simulink model "neuronchainv6"  (Simulink 7.6)
settings: Solver=ode45  StartTime=0.0  StopTime=300  RelTol=1e-3
values from neighbouring files (symbols this model uses):
  alpha = 0.8    [excneuroninit.m]
  beta = 0.05    [excneuroninit.m]
  inittime = 0.1    [excneuroninit.m]
  sensoryamp = 0.5    [excneuroninit.m]
  sigslopef = 1    [excneuroninit.m]
  sigslopei = 3    [excneuroninit.m]
  tau_s = 5    [excneuroninit.m]
libraries: simulink x500, neuronpoolibv3 x3
(part 1 of 18)
settings Model: Creator=root  LastModifiedBy=root
settings SolverCC: ZeroCrossAlgorithm=Adaptive

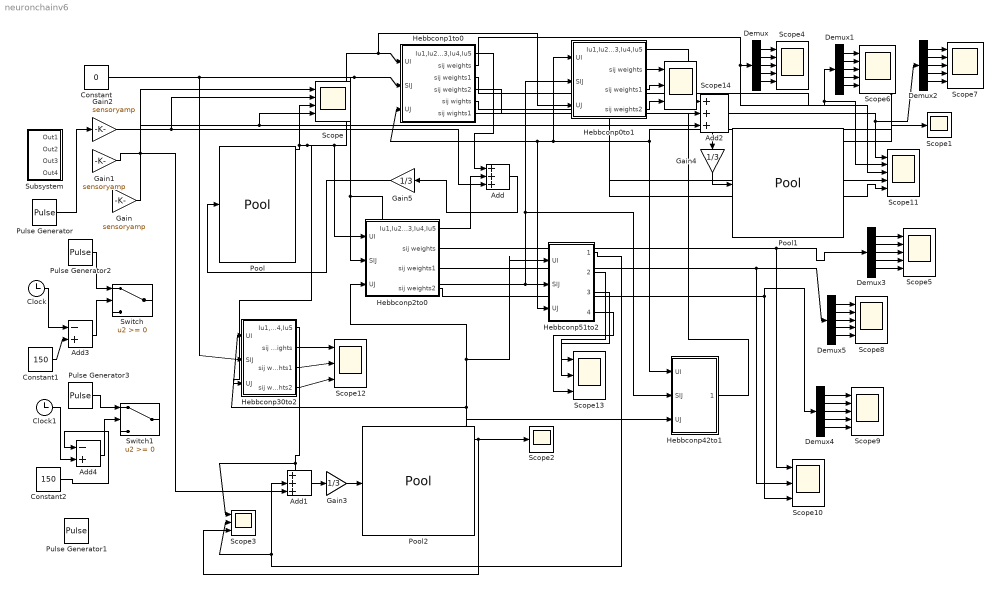
== system neuronchainv6 ==
  Add : Sum  Inputs=+++
  Add1 : Sum  Inputs=+++
  Add2 : Sum  Inputs=+++
  Add3 : Sum  Inputs=-+
  Add4 : Sum  Inputs=-+
  Clock : Clock
      settings: Decimation=10
  Clock1 : Clock
      settings: Decimation=10
  Constant : Constant  Value=0
  Constant1 : Constant  Value=150
  Constant2 : Constant  Value=150
  Demux{,1..5} (6 alike) : Demux  Outputs=5
  Gain : Gain  Gain=sensoryamp
  Gain1 : Gain  Gain=sensoryamp
  Gain2 : Gain  Gain=sensoryamp
  Gain3 : Gain  Gain=1/3
  Gain4 : Gain  Gain=1/3
  Gain5 : Gain  Gain=1/3
  Hebbconp0to1 : Subsystem
  Hebbconp1to0 : Subsystem
  Hebbconp2to0 : Subsystem
  Hebbconp30to2 : Subsystem
  Hebbconp42to1 : Subsystem
  Hebbconp51to2 : Subsystem
  Pool : neuronpoolibv3/Pool  SystemSampleTime=-1
  Pool1 : neuronpoolibv3/Pool  SystemSampleTime=-1
  Pool2 : neuronpoolibv3/Pool  SystemSampleTime=-1
  Pulse Generator : DiscretePulseGenerator  PulseType=Time based  Period=1  PulseWidth=50
  Pulse Generator1 : DiscretePulseGenerator  PulseType=Time based  Period=1  PulseWidth=50  PhaseDelay=0.5
  Pulse Generator2 : DiscretePulseGenerator  PulseType=Time based  PulseWidth=25  PhaseDelay=1.35
  Pulse Generator3 : DiscretePulseGenerator  PulseType=Time based  PulseWidth=25  PhaseDelay=1.35
  Scope : Scope  NumInputPorts=4
      settings: TimeRange=100  YMin=-1~0~3.9~-1  YMax=1~0.5~4.3~1
  Scope1 : Scope
      settings: YMin=6.5  YMax=12.25
  Scope{3,10,12..14} (5 alike) : Scope  NumInputPorts=3
      Scope10 settings: YMin=0.0405~0.04075~0.04075  YMax=0.0435~0.04375~0.044  SaveName=ScopeData10
      Scope12 settings: YMin=0.3~0.3~0.3  YMax=0.75~0.7~0.7  SaveName=ScopeData12
      Scope13 settings: YMin=0.06~0.06~0.06  YMax=0.15~0.14~0.14  SaveName=ScopeData13
      Scope14 settings: TimeRange=300  YMin=0.166~0.1635~0.1625  YMax=0.1715~0.169~0.1675  SaveName=ScopeData14
      Scope3 settings: YMin=3.46~3.4525~3.9  YMax=3.51~3.4825~4.1  SaveName=ScopeData3
  Scope{4..9,11} (7 alike) : Scope  NumInputPorts=5
      Scope11 settings: YMin=0.0053~0.0054~0.0054~-5~-5  YMax=0.0064~0.0065~0.0065~5~5  SaveName=ScopeData11
      Scope4 settings: YMin=0.177~0.162~0.1565~0.162~0.177  YMax=0.183~0.166~0.1605~0.166~0.183  SaveName=ScopeData4
      Scope5 settings: YMin=0.177~0.162~0.1565~0.162~0.177  YMax=0.183~0.166~0.1605~0.166~0.183  SaveName=ScopeData5
      Scope6 settings: YMin=0.567164~0.567164~0.567164~-5~-5  YMax=0.626866~0.626866~0.626866~5~5  SaveName=ScopeData6
      Scope7 settings: YMin=0.567164~0.567164~0.567164~-5~-5  YMax=0.626866~0.626866~0.626866~5~5  SaveName=ScopeData7
      Scope8 settings: YMin=0.171~0.14425~0.13725~0.14425~0.171  YMax=0.175~0.14625~0.13925~0.14625~0.175  SaveName=ScopeData8
      Scope9 settings: YMin=0.06~0.06~0.06~0.06~0.06  YMax=0.15~0.14~0.14~0.14~0.15  SaveName=ScopeData9
  Scope2 : Scope
      settings: SaveName=ScopeData2
  Subsystem : Subsystem
  Switch : Switch
  Switch1 : Switch
  wires:
  Pool/1 -> Hebbconp1to0/1(UI), Hebbconp0to1/3(UJ), Hebbconp2to0/1(UI), Hebbconp30to2/3(UJ), Scope/3
  Pool1/1 -> Hebbconp1to0/3(UJ), Hebbconp51to2/3(UJ), Hebbconp0to1/1(UI), Hebbconp42to1/1(UI), Scope1/1
  Pool2/1 -> Hebbconp2to0/3(UJ), Hebbconp51to2/1(UI), Hebbconp30to2/1(UI), Hebbconp42to1/3(UJ), Scope2/1, Scope3/3
  Hebbconp1to0/1(Iu1,Iu2,Iu3,Iu4,Iu5) -> Add/1
  Add/1 -> Gain5/1
  Hebbconp51to2/1(Iu1,Iu2,Iu3,Iu4,Iu5) -> Add1/2, Scope3/2
  Hebbconp30to2/1(Iu1,Iu2,Iu3,Iu4,Iu5) -> Add1/1, Scope3/1
  Add1/1 -> Gain3/1
  Hebbconp42to1/1(Iu1,Iu2,Iu3,Iu4,Iu5) -> Add2/2
  Add2/1 -> Gain4/1
  Constant/1 -> Hebbconp1to0/2(SIJ), Hebbconp42to1/2(SIJ), Hebbconp0to1/2(SIJ), Hebbconp51to2/2(SIJ), Hebbconp2to0/2(SIJ), Hebbconp30to2/2(SIJ)
  Hebbconp2to0/1(Iu1,Iu2,Iu3,Iu4,Iu5) -> Add/2
  Hebbconp2to0/2(sij weights) -> Demux3/1, Scope10/1
  Hebbconp2to0/3(sij weights1) -> Demux5/1, Scope10/2
  Hebbconp2to0/4(sij weights2) -> Demux4/1, Scope10/3
  Gain/1 -> Add2/3, Scope/4
  Gain1/1 -> Add1/3, Scope/1
  Gain2/1 -> Add/3, Scope/2
  Demux/1 -> Scope4/1
  Demux/2 -> Scope4/2
  Demux/3 -> Scope4/3
  Demux/4 -> Scope4/4
  Demux/5 -> Scope4/5
  Hebbconp1to0/2(sij weights) -> Demux/1, Scope11/3
  Demux1/1 -> Scope6/1
  Demux1/2 -> Scope6/2
  Demux1/3 -> Scope6/3
  Demux1/4 -> Scope6/4
  Demux1/5 -> Scope6/5
  Hebbconp1to0/3(sij weights1) -> Demux1/1, Scope11/2
  Demux2/1 -> Scope7/1
  Demux2/2 -> Scope7/2
  Demux2/3 -> Scope7/3
  Demux2/4 -> Scope7/4
  Demux2/5 -> Scope7/5
  Hebbconp1to0/4(sij weights2) -> Demux2/1, Scope11/1
  Demux5/1 -> Scope8/1
  Demux5/2 -> Scope8/2
  Demux5/3 -> Scope8/3
  Demux5/4 -> Scope8/4
  Demux5/5 -> Scope8/5
  Demux3/1 -> Scope5/1
  Demux3/2 -> Scope5/2
  Demux3/3 -> Scope5/3
  Demux3/4 -> Scope5/4
  Demux3/5 -> Scope5/5
  Demux4/1 -> Scope9/1
  Demux4/2 -> Scope9/2
  Demux4/3 -> Scope9/3
  Demux4/4 -> Scope9/4
  Demux4/5 -> Scope9/5
  Hebbconp1to0/5(sij wights) -> Scope11/4
  Hebbconp1to0/6(sij wights1) -> Scope11/5
  Hebbconp30to2/2(sij weights) -> Scope12/1
  Hebbconp30to2/3(sij weights1) -> Scope12/2
  Hebbconp30to2/4(sij weights2) -> Scope12/3
  Hebbconp51to2/2(sij weights) -> Scope13/1
  Hebbconp51to2/3(sij weights1) -> Scope13/2
  Hebbconp51to2/4(sij weights2) -> Scope13/3
  Hebbconp0to1/1(Iu1,Iu2,Iu3,Iu4,Iu5) -> Add2/1
  Hebbconp0to1/2(sij weights) -> Scope14/1
  Hebbconp0to1/3(sij weights1) -> Scope14/2
  Hebbconp0to1/4(sij weights2) -> Scope14/3
  Gain5/1 -> Pool/1
  Gain3/1 -> Pool2/1
  Gain4/1 -> Pool1/1
  Clock/1 -> Add3/1
  Constant1/1 -> Add3/2
  Add3/1 -> Switch/2
  Pulse Generator/1 -> Gain2/1
  Add4/1 -> Switch1/2
  Clock1/1 -> Add4/2
  Constant2/1 -> Add4/1
  Pulse Generator2/1 -> Switch/1
  Pulse Generator3/1 -> Switch1/1

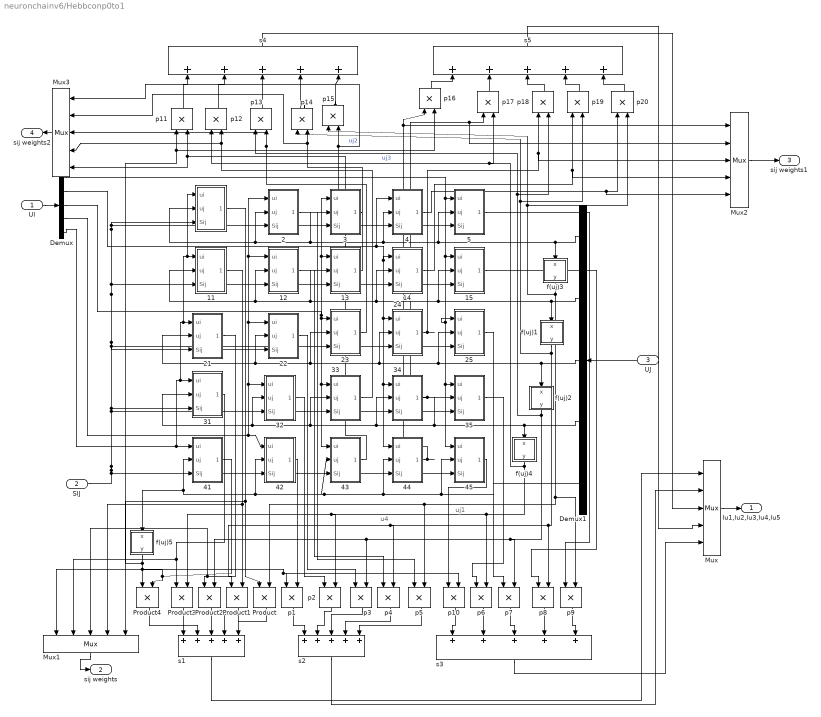
== system neuronchainv6/Hebbconp0to1 ==
  note: uj1
  note: u4
  UI : Inport
  SIJ : Inport  Port=2
  UJ : Inport  Port=3
  " " : Subsystem
  " 2" : Subsystem
  11 : Subsystem
  12 : Subsystem
  13 : Subsystem
  14 : Subsystem
  15 : Subsystem
  21 : Subsystem
  22 : Subsystem
  23 : Subsystem
  24 : Subsystem
  25 : Subsystem
  3 : Subsystem
  31 : Subsystem
  32 : Subsystem
  33 : Subsystem
  34 : Subsystem
  35 : Subsystem
  4 : Subsystem
  41 : Subsystem
  42 : Subsystem
  43 : Subsystem
  44 : Subsystem
  45 : Subsystem
  5 : Subsystem
  Demux : Demux  Outputs=5
  Demux1 : Demux  Outputs=5
  Mux{,1..3} (4 alike) : Mux  Inputs=5
  Product{,1..4} (5 alike) : Product  RndMeth=Zero
  f(uj)1 : Subsystem  TreatAsAtomicUnit=on  mask{slope=sigslopef, offset=0.5}
      mask help: Created by Han, Cheol
      mask Display: plot([10 15 20 25 30 35 40 45 50], [0 0.01 0.1 0.2 0.5 0.8 0.9 0.99 1])
  f(uj)2 : Subsystem  TreatAsAtomicUnit=on  mask{slope=sigslopef, offset=0.5}
      mask help: Created by Han, Cheol
      mask Display: plot([10 15 20 25 30 35 40 45 50], [0 0.01 0.1 0.2 0.5 0.8 0.9 0.99 1])
  f(uj)3 : Subsystem  TreatAsAtomicUnit=on  mask{slope=sigslopef, offset=0.5}
      mask help: Created by Han, Cheol
      mask Display: plot([10 15 20 25 30 35 40 45 50], [0 0.01 0.1 0.2 0.5 0.8 0.9 0.99 1])
  f(uj)4 : Subsystem  TreatAsAtomicUnit=on  mask{slope=sigslopef, offset=0.5}
      mask help: Created by Han, Cheol
      mask Display: plot([10 15 20 25 30 35 40 45 50], [0 0.01 0.1 0.2 0.5 0.8 0.9 0.99 1])
  f(uj)5 : Subsystem  TreatAsAtomicUnit=on  mask{slope=sigslopef, offset=0.5}
      mask help: Created by Han, Cheol
      mask Display: plot([10 15 20 25 30 35 40 45 50], [0 0.01 0.1 0.2 0.5 0.8 0.9 0.99 1])
  p{1..20} (20 alike) : Product  RndMeth=Zero
  s{1..5} (5 alike) : Sum  Inputs=+++++
  Iu1,Iu2,Iu3,Iu4,Iu5 : Outport
  sij weights : Outport  Port=2
  sij weights1 : Outport  Port=3
  sij weights2 : Outport  Port=4
  wires:
  Demux/1 -> 15/1(ui), 45/1(ui), 35/1(ui), 25/1(ui), 5/1(ui)
  Demux/2 -> 4/1(ui), 44/1(ui), 34/1(ui), 24/1(ui), 14/1(ui)
  Demux/3 -> 43/1(ui), 33/1(ui), 23/1(ui), 13/1(ui), 3/1(ui)
  Demux/4 -> 42/1(ui), 32/1(ui), 22/1(ui), 12/1(ui), " 2"/1(ui)
  Demux/5 -> 41/1(ui), 31/1(ui), 21/1(ui), 11/1(ui), " "/1(ui)
  Demux1/1 -> " "/2(uj), " 2"/2(uj), 3/2(uj), 4/2(uj), 5/2(uj), f(uj)3/1(x)
  Demux1/2 -> 11/2(uj), 12/2(uj), 13/2(uj), 14/2(uj), 15/2(uj), f(uj)1/1(x)
  Demux1/3 -> 25/2(uj), 21/2(uj), 22/2(uj), 23/2(uj), 24/2(uj), f(uj)2/1(x)
  Demux1/4 -> 31/2(uj), 32/2(uj), 33/2(uj), 34/2(uj), 35/2(uj), f(uj)4/1(x)
  Demux1/5 -> 42/2(uj), 41/2(uj), f(uj)5/1(x), 43/2(uj), 44/2(uj), 45/2(uj)
  " "/1(Out1) -> Product/1, Mux1/5
  11/1(Out1) -> Product1/2, Mux1/4
  41/1(Out1) -> Product4/2, Mux1/1
  21/1(Out1) -> Product2/1, Mux1/3
  31/1(Out1) -> Product3/1, Mux1/2
  f(uj)3/1(y) -> Product/2, p5/2, p9/2, p15/1, p20/2
  f(uj)1/1(y) -> Product1/1, p4/2, p8/2, p14/1, p19/2  "uj2"
  f(uj)2/1(y) -> Product2/2, p3/2, p7/2, p13/1, p18/2  "uj3"
  f(uj)4/1(y) -> Product3/2, p2/2, p6/2, p17/2, p12/1
  " 2"/1(Out1) -> p5/1
  12/1(Out1) -> p4/1
  22/1(Out1) -> p3/1
  32/1(Out1) -> p2/1
  42/1(Out1) -> p1/2
  f(uj)5/1(y) -> Product4/1, p1/1, p10/2, p11/1, p16/2
  5/1(Out1) -> p9/1
  15/1(Out1) -> p8/1
  25/1(Out1) -> p7/1
  35/1(Out1) -> p6/1
  45/1(Out1) -> p10/1
  3/1(Out1) -> p15/2, Mux3/1
  13/1(Out1) -> p14/2, Mux3/2
  23/1(Out1) -> p13/2, Mux3/3
  33/1(Out1) -> p12/2, Mux3/4
  43/1(Out1) -> p11/2, Mux3/5
  p15/1 -> s4/5
  p11/1 -> s4/1
  p12/1 -> s4/2
  p13/1 -> s4/3
  p14/1 -> s4/4
  UI/1 -> Demux/1
  4/1(Out1) -> p20/1, Mux2/5
  SIJ/1 -> 41/3(Sij), 21/3(Sij), 11/3(Sij), " "/3(Sij), " 2"/3(Sij), 3/3(Sij), 4/3(Sij), 5/3(Sij), 13/3(Sij), 14/3(Sij), 15/3(Sij), 12/3(Sij), 22/3(Sij), 23/3(Sij), 24/3(Sij), 25/3(Sij), 31/3(Sij), 33/3(Sij), 34/3(Sij), 35/3(Sij), 32/3(Sij), 42/3(Sij), 43/3(Sij), 44/3(Sij), 45/3(Sij)
  14/1(Out1) -> p19/1, Mux2/4
  24/1(Out1) -> p18/1, Mux2/3
  UJ/1 -> Demux1/1
  34/1(Out1) -> p17/1, Mux2/2
  44/1(Out1) -> p16/1, Mux2/1
  Product/1 -> s1/5
  Product1/1 -> s1/4
  Product2/1 -> s1/3
  Product3/1 -> s1/2
  Product4/1 -> s1/1
  p1/1 -> s2/1
  p10/1 -> s3/1
  p2/1 -> s2/2
  p3/1 -> s2/3
  p4/1 -> s2/4
  p5/1 -> s2/5
  p6/1 -> s3/2
  p7/1 -> s3/3
  p8/1 -> s3/4
  p9/1 -> s3/5
  p16/1 -> s5/1
  p17/1 -> s5/2
  p18/1 -> s5/3
  p19/1 -> s5/4
  p20/1 -> s5/5
  s4/1 -> Mux/3
  s1/1 -> Mux/1
  s2/1 -> Mux/2
  s3/1 -> Mux/5
  s5/1 -> Mux/4
  Mux/1 -> Iu1,Iu2,Iu3,Iu4,Iu5/1
  Mux1/1 -> sij weights/1
  Mux2/1 -> sij weights1/1
  Mux3/1 -> sij weights2/1

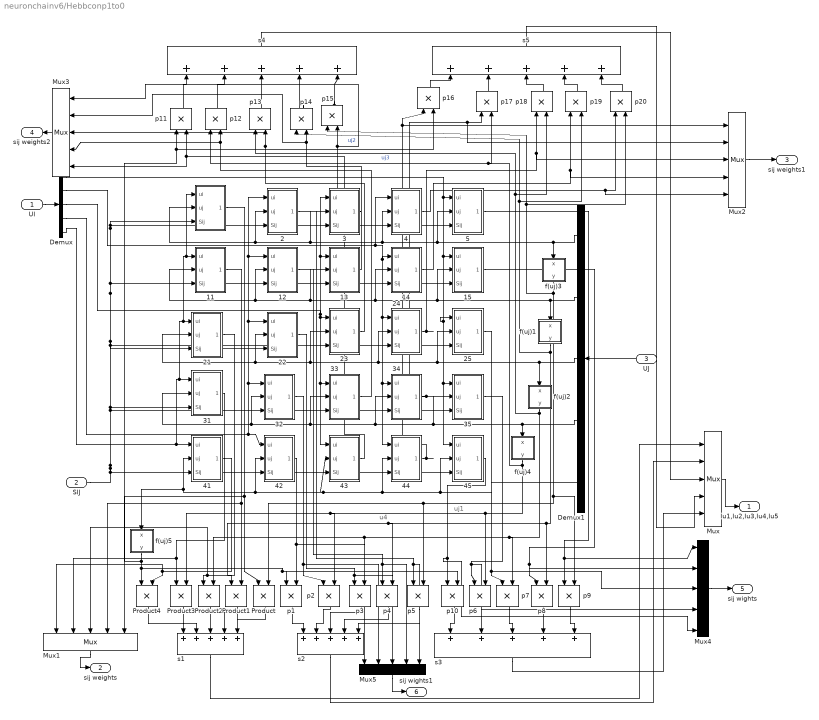
== system neuronchainv6/Hebbconp1to0 ==
  note: uj1
  note: u4
  UI : Inport
  SIJ : Inport  Port=2
  UJ : Inport  Port=3
  " " : Subsystem
  " 2" : Subsystem
  11 : Subsystem
  12 : Subsystem
  13 : Subsystem
  14 : Subsystem
  15 : Subsystem
  21 : Subsystem
  22 : Subsystem
  23 : Subsystem
  24 : Subsystem
  25 : Subsystem
  3 : Subsystem
  31 : Subsystem
  32 : Subsystem
  33 : Subsystem
  34 : Subsystem
  35 : Subsystem
  4 : Subsystem
  41 : Subsystem
  42 : Subsystem
  43 : Subsystem
  44 : Subsystem
  45 : Subsystem
  5 : Subsystem
  Demux : Demux  Outputs=5
  Demux1 : Demux  Outputs=5
  Mux{,1..5} (6 alike) : Mux  Inputs=5
  Product{,1..4} (5 alike) : Product  RndMeth=Zero
  f(uj)1 : Subsystem  TreatAsAtomicUnit=on  mask{slope=sigslopef, offset=0.5}
      mask help: Created by Han, Cheol
      mask Display: plot([10 15 20 25 30 35 40 45 50], [0 0.01 0.1 0.2 0.5 0.8 0.9 0.99 1])
  f(uj)2 : Subsystem  TreatAsAtomicUnit=on  mask{slope=sigslopef, offset=0.5}
      mask help: Created by Han, Cheol
      mask Display: plot([10 15 20 25 30 35 40 45 50], [0 0.01 0.1 0.2 0.5 0.8 0.9 0.99 1])
  f(uj)3 : Subsystem  TreatAsAtomicUnit=on  mask{slope=sigslopef, offset=0.5}
      mask help: Created by Han, Cheol
      mask Display: plot([10 15 20 25 30 35 40 45 50], [0 0.01 0.1 0.2 0.5 0.8 0.9 0.99 1])
  f(uj)4 : Subsystem  TreatAsAtomicUnit=on  mask{slope=sigslopef, offset=0.5}
      mask help: Created by Han, Cheol
      mask Display: plot([10 15 20 25 30 35 40 45 50], [0 0.01 0.1 0.2 0.5 0.8 0.9 0.99 1])
  f(uj)5 : Subsystem  TreatAsAtomicUnit=on  mask{slope=sigslopef, offset=0.5}
      mask help: Created by Han, Cheol
      mask Display: plot([10 15 20 25 30 35 40 45 50], [0 0.01 0.1 0.2 0.5 0.8 0.9 0.99 1])
  p{1..20} (20 alike) : Product  RndMeth=Zero
  s{1..5} (5 alike) : Sum  Inputs=+++++
  Iu1,Iu2,Iu3,Iu4,Iu5 : Outport
  sij weights : Outport  Port=2
  sij weights1 : Outport  Port=3
  sij weights2 : Outport  Port=4
  sij wights : Outport  Port=5
  sij wights1 : Outport  Port=6
  wires:
  Demux/1 -> 15/1(ui), 45/1(ui), 35/1(ui), 25/1(ui), 5/1(ui)
  Demux/2 -> 4/1(ui), 44/1(ui), 34/1(ui), 24/1(ui), 14/1(ui)
  Demux/3 -> 43/1(ui), 33/1(ui), 23/1(ui), 13/1(ui), 3/1(ui)
  Demux/4 -> 42/1(ui), 32/1(ui), 22/1(ui), 12/1(ui), " 2"/1(ui)
  Demux/5 -> 41/1(ui), 31/1(ui), 21/1(ui), 11/1(ui), " "/1(ui)
  Demux1/1 -> " "/2(uj), " 2"/2(uj), 3/2(uj), 4/2(uj), 5/2(uj), f(uj)3/1(x)
  Demux1/2 -> 11/2(uj), 12/2(uj), 13/2(uj), 14/2(uj), 15/2(uj), f(uj)1/1(x)
  Demux1/3 -> 25/2(uj), 21/2(uj), 22/2(uj), 23/2(uj), 24/2(uj), f(uj)2/1(x)
  Demux1/4 -> 31/2(uj), 32/2(uj), 33/2(uj), 34/2(uj), 35/2(uj), f(uj)4/1(x)
  Demux1/5 -> 42/2(uj), 41/2(uj), f(uj)5/1(x), 43/2(uj), 44/2(uj), 45/2(uj)
  " "/1(Out1) -> Product/1, Mux1/5
  11/1(Out1) -> Product1/2, Mux1/4
  41/1(Out1) -> Product4/2, Mux1/1
  21/1(Out1) -> Product2/1, Mux1/3
  31/1(Out1) -> Product3/1, Mux1/2
  f(uj)3/1(y) -> Product/2, p5/2, p9/2, p15/1, p20/2
  f(uj)1/1(y) -> Product1/1, p4/2, p8/2, p14/1, p19/2  "uj2"
  f(uj)2/1(y) -> Product2/2, p3/2, p7/2, p13/1, p18/2  "uj3"
  f(uj)4/1(y) -> Product3/2, p2/2, p6/2, p17/2, p12/1
  " 2"/1(Out1) -> p5/1, Mux5/5
  12/1(Out1) -> p4/1, Mux5/4
  22/1(Out1) -> p3/1, Mux5/3
  32/1(Out1) -> p2/1, Mux5/2
  42/1(Out1) -> p1/2, Mux5/1
  f(uj)5/1(y) -> Product4/1, p1/1, p10/2, p11/1, p16/2
  5/1(Out1) -> p9/1, Mux4/1
  15/1(Out1) -> p8/1, Mux4/2
  25/1(Out1) -> p7/1, Mux4/3
  35/1(Out1) -> p6/1, Mux4/4
  45/1(Out1) -> p10/1, Mux4/5
  3/1(Out1) -> p15/2, Mux3/1
  13/1(Out1) -> p14/2, Mux3/2
  23/1(Out1) -> p13/2, Mux3/3
  33/1(Out1) -> p12/2, Mux3/4
  43/1(Out1) -> p11/2, Mux3/5
  p15/1 -> s4/5
  p11/1 -> s4/1
  p12/1 -> s4/2
  p13/1 -> s4/3
  p14/1 -> s4/4
  UI/1 -> Demux/1
  4/1(Out1) -> p20/1, Mux2/5
  SIJ/1 -> 41/3(Sij), 21/3(Sij), 11/3(Sij), " "/3(Sij), " 2"/3(Sij), 3/3(Sij), 4/3(Sij), 5/3(Sij), 13/3(Sij), 14/3(Sij), 15/3(Sij), 12/3(Sij), 22/3(Sij), 23/3(Sij), 24/3(Sij), 25/3(Sij), 31/3(Sij), 33/3(Sij), 34/3(Sij), 35/3(Sij), 32/3(Sij), 42/3(Sij), 43/3(Sij), 44/3(Sij), 45/3(Sij)
  14/1(Out1) -> p19/1, Mux2/4
  24/1(Out1) -> p18/1, Mux2/3
  UJ/1 -> Demux1/1
  34/1(Out1) -> p17/1, Mux2/2
  44/1(Out1) -> p16/1, Mux2/1
  Product/1 -> s1/5
  Product1/1 -> s1/4
  Product2/1 -> s1/3
  Product3/1 -> s1/2
  Product4/1 -> s1/1
  p1/1 -> s2/1
  p10/1 -> s3/1
  p2/1 -> s2/2
  p3/1 -> s2/3
  p4/1 -> s2/4
  p5/1 -> s2/5
  p6/1 -> s3/2
  p7/1 -> s3/3
  p8/1 -> s3/4
  p9/1 -> s3/5
  p16/1 -> s5/1
  p17/1 -> s5/2
  p18/1 -> s5/3
  p19/1 -> s5/4
  p20/1 -> s5/5
  s4/1 -> Mux/3
  s1/1 -> Mux/1
  s2/1 -> Mux/2
  s3/1 -> Mux/5
  s5/1 -> Mux/4
  Mux/1 -> Iu1,Iu2,Iu3,Iu4,Iu5/1
  Mux1/1 -> sij weights/1
  Mux2/1 -> sij weights1/1
  Mux3/1 -> sij weights2/1
  Mux4/1 -> sij wights/1
  Mux5/1 -> sij wights1/1

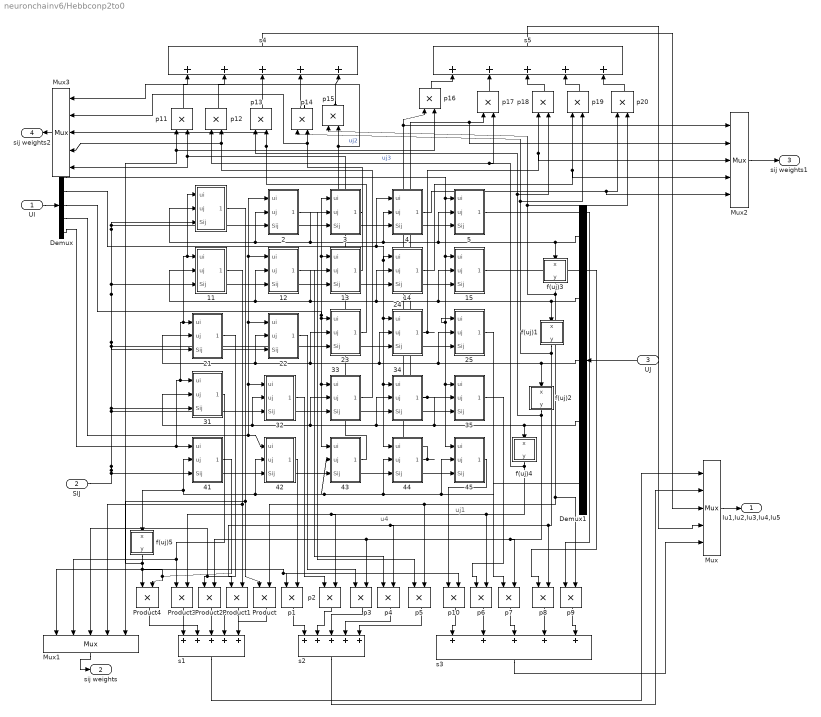
== system neuronchainv6/Hebbconp2to0 ==
  note: uj1
  note: u4
  UI : Inport
  SIJ : Inport  Port=2
  UJ : Inport  Port=3
  " " : Subsystem
  " 2" : Subsystem
  11 : Subsystem
  12 : Subsystem
  13 : Subsystem
  14 : Subsystem
  15 : Subsystem
  21 : Subsystem
  22 : Subsystem
  23 : Subsystem
  24 : Subsystem
  25 : Subsystem
  3 : Subsystem
  31 : Subsystem
  32 : Subsystem
  33 : Subsystem
  34 : Subsystem
  35 : Subsystem
  4 : Subsystem
  41 : Subsystem
  42 : Subsystem
  43 : Subsystem
  44 : Subsystem
  45 : Subsystem
  5 : Subsystem
  Demux : Demux  Outputs=5
  Demux1 : Demux  Outputs=5
  Mux{,1..3} (4 alike) : Mux  Inputs=5
  Product{,1..4} (5 alike) : Product  RndMeth=Zero
  f(uj)1 : Subsystem  TreatAsAtomicUnit=on  mask{slope=sigslopef, offset=0.5}
      mask help: Created by Han, Cheol
      mask Display: plot([10 15 20 25 30 35 40 45 50], [0 0.01 0.1 0.2 0.5 0.8 0.9 0.99 1])
  f(uj)2 : Subsystem  TreatAsAtomicUnit=on  mask{slope=sigslopef, offset=0.5}
      mask help: Created by Han, Cheol
      mask Display: plot([10 15 20 25 30 35 40 45 50], [0 0.01 0.1 0.2 0.5 0.8 0.9 0.99 1])
  f(uj)3 : Subsystem  TreatAsAtomicUnit=on  mask{slope=sigslopef, offset=0.5}
      mask help: Created by Han, Cheol
      mask Display: plot([10 15 20 25 30 35 40 45 50], [0 0.01 0.1 0.2 0.5 0.8 0.9 0.99 1])
  f(uj)4 : Subsystem  TreatAsAtomicUnit=on  mask{slope=sigslopef, offset=0.5}
      mask help: Created by Han, Cheol
      mask Display: plot([10 15 20 25 30 35 40 45 50], [0 0.01 0.1 0.2 0.5 0.8 0.9 0.99 1])
  f(uj)5 : Subsystem  TreatAsAtomicUnit=on  mask{slope=sigslopef, offset=0.5}
      mask help: Created by Han, Cheol
      mask Display: plot([10 15 20 25 30 35 40 45 50], [0 0.01 0.1 0.2 0.5 0.8 0.9 0.99 1])
  p{1..20} (20 alike) : Product  RndMeth=Zero
  s{1..5} (5 alike) : Sum  Inputs=+++++
  Iu1,Iu2,Iu3,Iu4,Iu5 : Outport
  sij weights : Outport  Port=2
  sij weights1 : Outport  Port=3
  sij weights2 : Outport  Port=4
  wires:
  Demux/1 -> 15/1(ui), 45/1(ui), 35/1(ui), 25/1(ui), 5/1(ui)
  Demux/2 -> 4/1(ui), 44/1(ui), 34/1(ui), 24/1(ui), 14/1(ui)
  Demux/3 -> 43/1(ui), 33/1(ui), 23/1(ui), 13/1(ui), 3/1(ui)
  Demux/4 -> 42/1(ui), 32/1(ui), 22/1(ui), 12/1(ui), " 2"/1(ui)
  Demux/5 -> 41/1(ui), 31/1(ui), 21/1(ui), 11/1(ui), " "/1(ui)
  Demux1/1 -> " "/2(uj), " 2"/2(uj), 3/2(uj), 4/2(uj), 5/2(uj), f(uj)3/1(x)
  Demux1/2 -> 11/2(uj), 12/2(uj), 13/2(uj), 14/2(uj), 15/2(uj), f(uj)1/1(x)
  Demux1/3 -> 25/2(uj), 21/2(uj), 22/2(uj), 23/2(uj), 24/2(uj), f(uj)2/1(x)
  Demux1/4 -> 31/2(uj), 32/2(uj), 33/2(uj), 34/2(uj), 35/2(uj), f(uj)4/1(x)
  Demux1/5 -> 42/2(uj), 41/2(uj), f(uj)5/1(x), 43/2(uj), 44/2(uj), 45/2(uj)
  " "/1(Out1) -> Product/1, Mux1/5
  11/1(Out1) -> Product1/2, Mux1/4
  41/1(Out1) -> Product4/2, Mux1/1
  21/1(Out1) -> Product2/1, Mux1/3
  31/1(Out1) -> Product3/1, Mux1/2
  f(uj)3/1(y) -> Product/2, p5/2, p9/2, p15/1, p20/2
  f(uj)1/1(y) -> Product1/1, p4/2, p8/2, p14/1, p19/2  "uj2"
  f(uj)2/1(y) -> Product2/2, p3/2, p7/2, p13/1, p18/2  "uj3"
  f(uj)4/1(y) -> Product3/2, p2/2, p6/2, p17/2, p12/1
  " 2"/1(Out1) -> p5/1
  12/1(Out1) -> p4/1
  22/1(Out1) -> p3/1
  32/1(Out1) -> p2/1
  42/1(Out1) -> p1/2
  f(uj)5/1(y) -> Product4/1, p1/1, p10/2, p11/1, p16/2
  5/1(Out1) -> p9/1
  15/1(Out1) -> p8/1
  25/1(Out1) -> p7/1
  35/1(Out1) -> p6/1
  45/1(Out1) -> p10/1
  3/1(Out1) -> p15/2, Mux3/1
  13/1(Out1) -> p14/2, Mux3/2
  23/1(Out1) -> p13/2, Mux3/3
  33/1(Out1) -> p12/2, Mux3/4
  43/1(Out1) -> p11/2, Mux3/5
  p15/1 -> s4/5
  p11/1 -> s4/1
  p12/1 -> s4/2
  p13/1 -> s4/3
  p14/1 -> s4/4
  UI/1 -> Demux/1
  4/1(Out1) -> p20/1, Mux2/5
  SIJ/1 -> 41/3(Sij), 21/3(Sij), 11/3(Sij), " "/3(Sij), " 2"/3(Sij), 3/3(Sij), 4/3(Sij), 5/3(Sij), 13/3(Sij), 14/3(Sij), 15/3(Sij), 12/3(Sij), 22/3(Sij), 23/3(Sij), 24/3(Sij), 25/3(Sij), 31/3(Sij), 33/3(Sij), 34/3(Sij), 35/3(Sij), 32/3(Sij), 42/3(Sij), 43/3(Sij), 44/3(Sij), 45/3(Sij)
  14/1(Out1) -> p19/1, Mux2/4
  24/1(Out1) -> p18/1, Mux2/3
  UJ/1 -> Demux1/1
  34/1(Out1) -> p17/1, Mux2/2
  44/1(Out1) -> p16/1, Mux2/1
  Product/1 -> s1/5
  Product1/1 -> s1/4
  Product2/1 -> s1/3
  Product3/1 -> s1/2
  Product4/1 -> s1/1
  p1/1 -> s2/1
  p10/1 -> s3/1
  p2/1 -> s2/2
  p3/1 -> s2/3
  p4/1 -> s2/4
  p5/1 -> s2/5
  p6/1 -> s3/2
  p7/1 -> s3/3
  p8/1 -> s3/4
  p9/1 -> s3/5
  p16/1 -> s5/1
  p17/1 -> s5/2
  p18/1 -> s5/3
  p19/1 -> s5/4
  p20/1 -> s5/5
  s4/1 -> Mux/3
  s1/1 -> Mux/1
  s2/1 -> Mux/2
  s3/1 -> Mux/5
  s5/1 -> Mux/4
  Mux/1 -> Iu1,Iu2,Iu3,Iu4,Iu5/1
  Mux1/1 -> sij weights/1
  Mux2/1 -> sij weights1/1
  Mux3/1 -> sij weights2/1

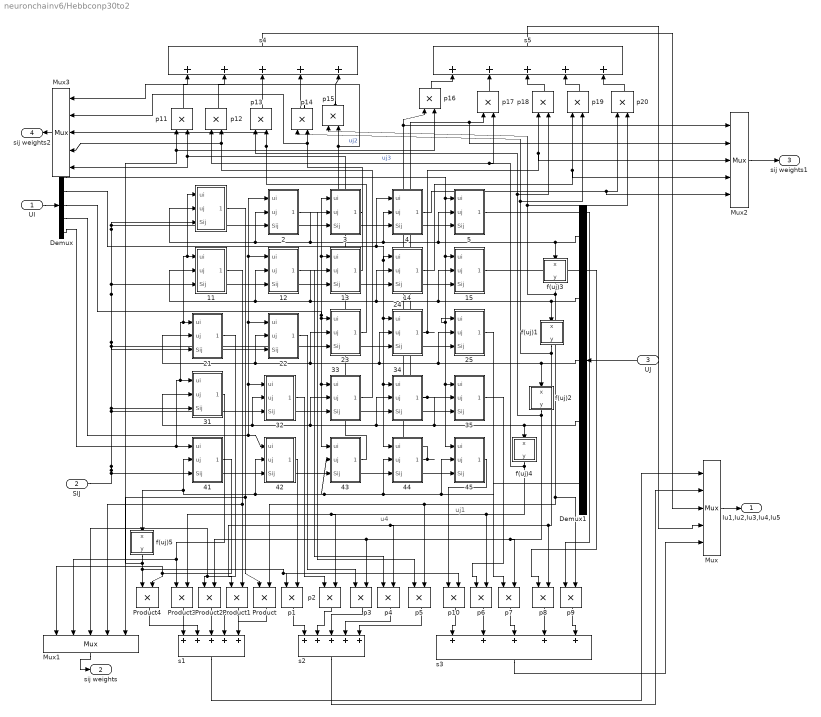
== system neuronchainv6/Hebbconp30to2 ==
  note: uj1
  note: u4
  UI : Inport
  SIJ : Inport  Port=2
  UJ : Inport  Port=3
  " " : Subsystem
  " 2" : Subsystem
  11 : Subsystem
  12 : Subsystem
  13 : Subsystem
  14 : Subsystem
  15 : Subsystem
  21 : Subsystem
  22 : Subsystem
  23 : Subsystem
  24 : Subsystem
  25 : Subsystem
  3 : Subsystem
  31 : Subsystem
  32 : Subsystem
  33 : Subsystem
  34 : Subsystem
  35 : Subsystem
  4 : Subsystem
  41 : Subsystem
  42 : Subsystem
  43 : Subsystem
  44 : Subsystem
  45 : Subsystem
  5 : Subsystem
  Demux : Demux  Outputs=5
  Demux1 : Demux  Outputs=5
  Mux{,1..3} (4 alike) : Mux  Inputs=5
  Product{,1..4} (5 alike) : Product  RndMeth=Zero
  f(uj)1 : Subsystem  TreatAsAtomicUnit=on  mask{slope=sigslopef, offset=0.5}
      mask help: Created by Han, Cheol
      mask Display: plot([10 15 20 25 30 35 40 45 50], [0 0.01 0.1 0.2 0.5 0.8 0.9 0.99 1])
  f(uj)2 : Subsystem  TreatAsAtomicUnit=on  mask{slope=sigslopef, offset=0.5}
      mask help: Created by Han, Cheol
      mask Display: plot([10 15 20 25 30 35 40 45 50], [0 0.01 0.1 0.2 0.5 0.8 0.9 0.99 1])
  f(uj)3 : Subsystem  TreatAsAtomicUnit=on  mask{slope=sigslopef, offset=0.5}
      mask help: Created by Han, Cheol
      mask Display: plot([10 15 20 25 30 35 40 45 50], [0 0.01 0.1 0.2 0.5 0.8 0.9 0.99 1])
  f(uj)4 : Subsystem  TreatAsAtomicUnit=on  mask{slope=sigslopef, offset=0.5}
      mask help: Created by Han, Cheol
      mask Display: plot([10 15 20 25 30 35 40 45 50], [0 0.01 0.1 0.2 0.5 0.8 0.9 0.99 1])
  f(uj)5 : Subsystem  TreatAsAtomicUnit=on  mask{slope=sigslopef, offset=0.5}
      mask help: Created by Han, Cheol
      mask Display: plot([10 15 20 25 30 35 40 45 50], [0 0.01 0.1 0.2 0.5 0.8 0.9 0.99 1])
  p{1..20} (20 alike) : Product  RndMeth=Zero
  s{1..5} (5 alike) : Sum  Inputs=+++++
  Iu1,Iu2,Iu3,Iu4,Iu5 : Outport
  sij weights : Outport  Port=2
  sij weights1 : Outport  Port=3
  sij weights2 : Outport  Port=4
  wires:
  Demux/1 -> 15/1(ui), 45/1(ui), 35/1(ui), 25/1(ui), 5/1(ui)
  Demux/2 -> 4/1(ui), 44/1(ui), 34/1(ui), 24/1(ui), 14/1(ui)
  Demux/3 -> 43/1(ui), 33/1(ui), 23/1(ui), 13/1(ui), 3/1(ui)
  Demux/4 -> 42/1(ui), 32/1(ui), 22/1(ui), 12/1(ui), " 2"/1(ui)
  Demux/5 -> 41/1(ui), 31/1(ui), 21/1(ui), 11/1(ui), " "/1(ui)
  Demux1/1 -> " "/2(uj), " 2"/2(uj), 3/2(uj), 4/2(uj), 5/2(uj), f(uj)3/1(x)
  Demux1/2 -> 11/2(uj), 12/2(uj), 13/2(uj), 14/2(uj), 15/2(uj), f(uj)1/1(x)
  Demux1/3 -> 25/2(uj), 21/2(uj), 22/2(uj), 23/2(uj), 24/2(uj), f(uj)2/1(x)
  Demux1/4 -> 31/2(uj), 32/2(uj), 33/2(uj), 34/2(uj), 35/2(uj), f(uj)4/1(x)
  Demux1/5 -> 42/2(uj), 41/2(uj), f(uj)5/1(x), 43/2(uj), 44/2(uj), 45/2(uj)
  " "/1(Out1) -> Product/1, Mux1/5
  11/1(Out1) -> Product1/2, Mux1/4
  41/1(Out1) -> Product4/2, Mux1/1
  21/1(Out1) -> Product2/1, Mux1/3
  31/1(Out1) -> Product3/1, Mux1/2
  f(uj)3/1(y) -> Product/2, p5/2, p9/2, p15/1, p20/2
  f(uj)1/1(y) -> Product1/1, p4/2, p8/2, p14/1, p19/2  "uj2"
  f(uj)2/1(y) -> Product2/2, p3/2, p7/2, p13/1, p18/2  "uj3"
  f(uj)4/1(y) -> Product3/2, p2/2, p6/2, p17/2, p12/1
  " 2"/1(Out1) -> p5/1
  12/1(Out1) -> p4/1
  22/1(Out1) -> p3/1
  32/1(Out1) -> p2/1
  42/1(Out1) -> p1/2
  f(uj)5/1(y) -> Product4/1, p1/1, p10/2, p11/1, p16/2
  5/1(Out1) -> p9/1
  15/1(Out1) -> p8/1
  25/1(Out1) -> p7/1
  35/1(Out1) -> p6/1
  45/1(Out1) -> p10/1
  3/1(Out1) -> p15/2, Mux3/1
  13/1(Out1) -> p14/2, Mux3/2
  23/1(Out1) -> p13/2, Mux3/3
  33/1(Out1) -> p12/2, Mux3/4
  43/1(Out1) -> p11/2, Mux3/5
  p15/1 -> s4/5
  p11/1 -> s4/1
  p12/1 -> s4/2
  p13/1 -> s4/3
  p14/1 -> s4/4
  UI/1 -> Demux/1
  4/1(Out1) -> p20/1, Mux2/5
  SIJ/1 -> 41/3(Sij), 21/3(Sij), 11/3(Sij), " "/3(Sij), " 2"/3(Sij), 3/3(Sij), 4/3(Sij), 5/3(Sij), 13/3(Sij), 14/3(Sij), 15/3(Sij), 12/3(Sij), 22/3(Sij), 23/3(Sij), 24/3(Sij), 25/3(Sij), 31/3(Sij), 33/3(Sij), 34/3(Sij), 35/3(Sij), 32/3(Sij), 42/3(Sij), 43/3(Sij), 44/3(Sij), 45/3(Sij)
  14/1(Out1) -> p19/1, Mux2/4
  24/1(Out1) -> p18/1, Mux2/3
  UJ/1 -> Demux1/1
  34/1(Out1) -> p17/1, Mux2/2
  44/1(Out1) -> p16/1, Mux2/1
  Product/1 -> s1/5
  Product1/1 -> s1/4
  Product2/1 -> s1/3
  Product3/1 -> s1/2
  Product4/1 -> s1/1
  p1/1 -> s2/1
  p10/1 -> s3/1
  p2/1 -> s2/2
  p3/1 -> s2/3
  p4/1 -> s2/4
  p5/1 -> s2/5
  p6/1 -> s3/2
  p7/1 -> s3/3
  p8/1 -> s3/4
  p9/1 -> s3/5
  p16/1 -> s5/1
  p17/1 -> s5/2
  p18/1 -> s5/3
  p19/1 -> s5/4
  p20/1 -> s5/5
  s4/1 -> Mux/3
  s1/1 -> Mux/1
  s2/1 -> Mux/2
  s3/1 -> Mux/5
  s5/1 -> Mux/4
  Mux/1 -> Iu1,Iu2,Iu3,Iu4,Iu5/1
  Mux1/1 -> sij weights/1
  Mux2/1 -> sij weights1/1
  Mux3/1 -> sij weights2/1

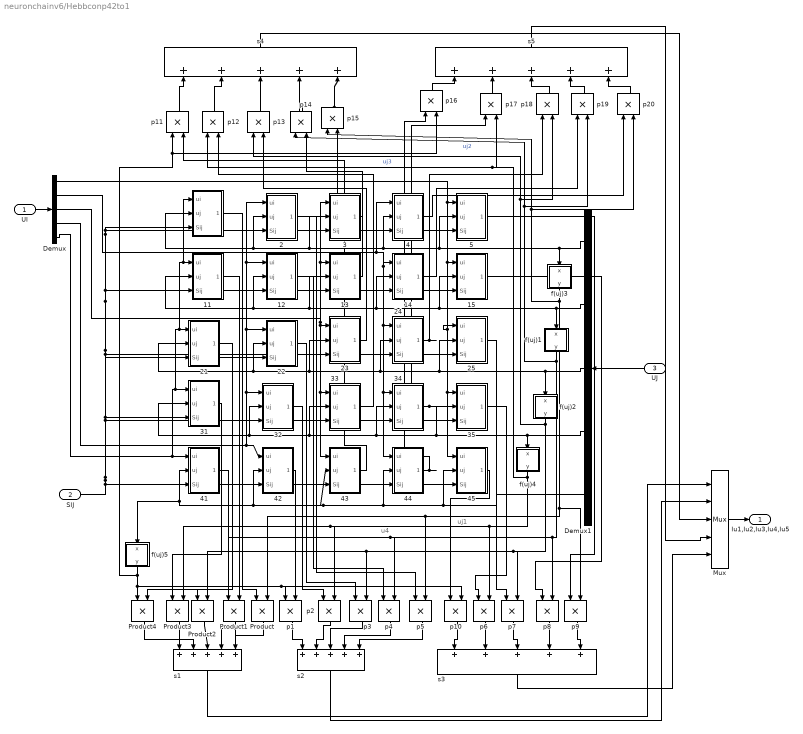
== system neuronchainv6/Hebbconp42to1 ==
  note: uj1
  note: u4
  UI : Inport
  SIJ : Inport  Port=2
  UJ : Inport  Port=3
  " " : Subsystem
  " 2" : Subsystem
  11 : Subsystem
  12 : Subsystem
  13 : Subsystem
  14 : Subsystem
  15 : Subsystem
  21 : Subsystem
  22 : Subsystem
  23 : Subsystem
  24 : Subsystem
  25 : Subsystem
  3 : Subsystem
  31 : Subsystem
  32 : Subsystem
  33 : Subsystem
  34 : Subsystem
  35 : Subsystem
  4 : Subsystem
  41 : Subsystem
  42 : Subsystem
  43 : Subsystem
  44 : Subsystem
  45 : Subsystem
  5 : Subsystem
  Demux : Demux  Outputs=5
  Demux1 : Demux  Outputs=5
  Mux : Mux  Inputs=5
  Product{,1..4} (5 alike) : Product  RndMeth=Zero
  f(uj)1 : Subsystem  TreatAsAtomicUnit=on  mask{slope=sigslopef, offset=0.5}
      mask help: Created by Han, Cheol
      mask Display: plot([10 15 20 25 30 35 40 45 50], [0 0.01 0.1 0.2 0.5 0.8 0.9 0.99 1])
  f(uj)2 : Subsystem  TreatAsAtomicUnit=on  mask{slope=sigslopef, offset=0.5}
      mask help: Created by Han, Cheol
      mask Display: plot([10 15 20 25 30 35 40 45 50], [0 0.01 0.1 0.2 0.5 0.8 0.9 0.99 1])
  f(uj)3 : Subsystem  TreatAsAtomicUnit=on  mask{slope=sigslopef, offset=0.5}
      mask help: Created by Han, Cheol
      mask Display: plot([10 15 20 25 30 35 40 45 50], [0 0.01 0.1 0.2 0.5 0.8 0.9 0.99 1])
  f(uj)4 : Subsystem  TreatAsAtomicUnit=on  mask{slope=sigslopef, offset=0.5}
      mask help: Created by Han, Cheol
      mask Display: plot([10 15 20 25 30 35 40 45 50], [0 0.01 0.1 0.2 0.5 0.8 0.9 0.99 1])
  f(uj)5 : Subsystem  TreatAsAtomicUnit=on  mask{slope=sigslopef, offset=0.5}
      mask help: Created by Han, Cheol
      mask Display: plot([10 15 20 25 30 35 40 45 50], [0 0.01 0.1 0.2 0.5 0.8 0.9 0.99 1])
  p{1..20} (20 alike) : Product  RndMeth=Zero
  s{1..5} (5 alike) : Sum  Inputs=+++++
  Iu1,Iu2,Iu3,Iu4,Iu5 : Outport
  wires:
  Demux/1 -> 15/1(ui), 45/1(ui), 35/1(ui), 25/1(ui), 5/1(ui)
  Demux/2 -> 4/1(ui), 44/1(ui), 34/1(ui), 24/1(ui), 14/1(ui)
  Demux/3 -> 43/1(ui), 33/1(ui), 23/1(ui), 13/1(ui), 3/1(ui)
  Demux/4 -> 42/1(ui), 32/1(ui), 22/1(ui), 12/1(ui), " 2"/1(ui)
  Demux/5 -> 41/1(ui), 31/1(ui), 21/1(ui), 11/1(ui), " "/1(ui)
  Demux1/1 -> " "/2(uj), " 2"/2(uj), 3/2(uj), 4/2(uj), 5/2(uj), f(uj)3/1(x)
  Demux1/2 -> 11/2(uj), 12/2(uj), 13/2(uj), 14/2(uj), 15/2(uj), f(uj)1/1(x)
  Demux1/3 -> 25/2(uj), 21/2(uj), 22/2(uj), 23/2(uj), 24/2(uj), f(uj)2/1(x)
  Demux1/4 -> 31/2(uj), 32/2(uj), 33/2(uj), 34/2(uj), 35/2(uj), f(uj)4/1(x)
  Demux1/5 -> 42/2(uj), 41/2(uj), f(uj)5/1(x), 43/2(uj), 44/2(uj), 45/2(uj)
  " "/1(Out1) -> Product/1
  11/1(Out1) -> Product1/2
  41/1(Out1) -> Product4/2
  21/1(Out1) -> Product2/1
  31/1(Out1) -> Product3/1
  f(uj)3/1(y) -> Product/2, p5/2, p9/2, p15/1, p20/2
  f(uj)1/1(y) -> Product1/1, p4/2, p8/2, p14/1, p19/2  "uj2"
  f(uj)2/1(y) -> Product2/2, p3/2, p7/2, p13/1, p18/2  "uj3"
  f(uj)4/1(y) -> Product3/2, p2/2, p6/2, p17/2, p12/1
  " 2"/1(Out1) -> p5/1
  12/1(Out1) -> p4/1
  22/1(Out1) -> p3/1
  32/1(Out1) -> p2/1
  42/1(Out1) -> p1/2
  f(uj)5/1(y) -> Product4/1, p1/1, p10/2, p11/1, p16/2
  5/1(Out1) -> p9/1
  15/1(Out1) -> p8/1
  25/1(Out1) -> p7/1
  35/1(Out1) -> p6/1
  45/1(Out1) -> p10/1
  3/1(Out1) -> p15/2
  13/1(Out1) -> p14/2
  23/1(Out1) -> p13/2
  33/1(Out1) -> p12/2
  43/1(Out1) -> p11/2
  p15/1 -> s4/5
  p11/1 -> s4/1
  p12/1 -> s4/2
  p13/1 -> s4/3
  p14/1 -> s4/4
  UI/1 -> Demux/1
  4/1(Out1) -> p20/1
  SIJ/1 -> 41/3(Sij), 21/3(Sij), 11/3(Sij), " "/3(Sij), " 2"/3(Sij), 3/3(Sij), 4/3(Sij), 5/3(Sij), 13/3(Sij), 14/3(Sij), 15/3(Sij), 12/3(Sij), 22/3(Sij), 23/3(Sij), 24/3(Sij), 25/3(Sij), 31/3(Sij), 33/3(Sij), 34/3(Sij), 35/3(Sij), 32/3(Sij), 42/3(Sij), 43/3(Sij), 44/3(Sij), 45/3(Sij)
  14/1(Out1) -> p19/1
  24/1(Out1) -> p18/1
  UJ/1 -> Demux1/1
  34/1(Out1) -> p17/1
  44/1(Out1) -> p16/1
  Product/1 -> s1/5
  Product1/1 -> s1/4
  Product2/1 -> s1/3
  Product3/1 -> s1/2
  Product4/1 -> s1/1
  p1/1 -> s2/1
  p10/1 -> s3/1
  p2/1 -> s2/2
  p3/1 -> s2/3
  p4/1 -> s2/4
  p5/1 -> s2/5
  p6/1 -> s3/2
  p7/1 -> s3/3
  p8/1 -> s3/4
  p9/1 -> s3/5
  p16/1 -> s5/1
  p17/1 -> s5/2
  p18/1 -> s5/3
  p19/1 -> s5/4
  p20/1 -> s5/5
  s4/1 -> Mux/3
  s1/1 -> Mux/1
  s2/1 -> Mux/2
  s3/1 -> Mux/5
  s5/1 -> Mux/4
  Mux/1 -> Iu1,Iu2,Iu3,Iu4,Iu5/1

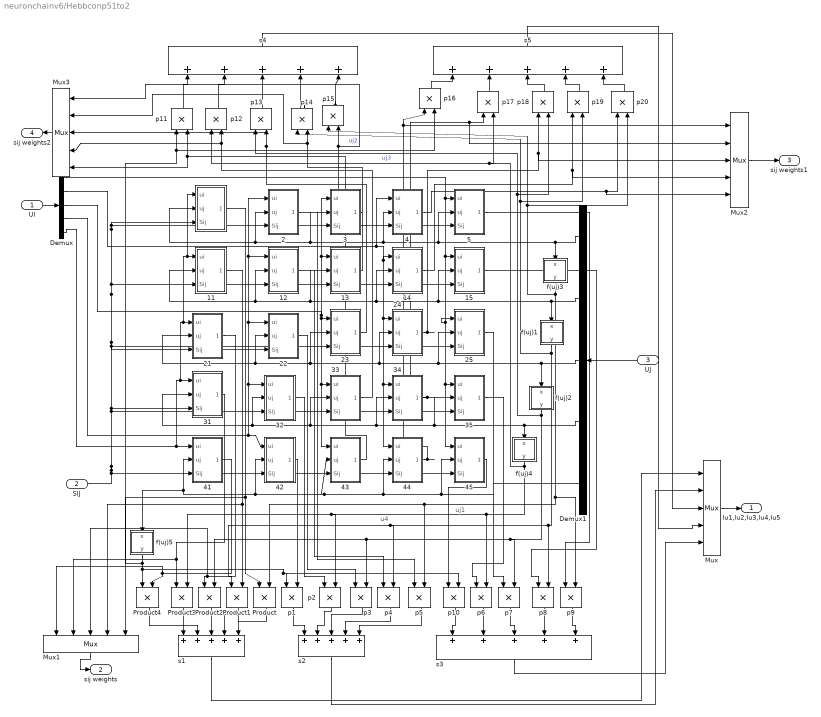
== system neuronchainv6/Hebbconp51to2 ==
  note: uj1
  note: u4
  UI : Inport
  SIJ : Inport  Port=2
  UJ : Inport  Port=3
  " " : Subsystem
  " 2" : Subsystem
  11 : Subsystem
  12 : Subsystem
  13 : Subsystem
  14 : Subsystem
  15 : Subsystem
  21 : Subsystem
  22 : Subsystem
  23 : Subsystem
  24 : Subsystem
  25 : Subsystem
  3 : Subsystem
  31 : Subsystem
  32 : Subsystem
  33 : Subsystem
  34 : Subsystem
  35 : Subsystem
  4 : Subsystem
  41 : Subsystem
  42 : Subsystem
  43 : Subsystem
  44 : Subsystem
  45 : Subsystem
  5 : Subsystem
  Demux : Demux  Outputs=5
  Demux1 : Demux  Outputs=5
  Mux{,1..3} (4 alike) : Mux  Inputs=5
  Product{,1..4} (5 alike) : Product  RndMeth=Zero
  f(uj)1 : Subsystem  TreatAsAtomicUnit=on  mask{slope=sigslopef, offset=0.5}
      mask help: Created by Han, Cheol
      mask Display: plot([10 15 20 25 30 35 40 45 50], [0 0.01 0.1 0.2 0.5 0.8 0.9 0.99 1])
  f(uj)2 : Subsystem  TreatAsAtomicUnit=on  mask{slope=sigslopef, offset=0.5}
      mask help: Created by Han, Cheol
      mask Display: plot([10 15 20 25 30 35 40 45 50], [0 0.01 0.1 0.2 0.5 0.8 0.9 0.99 1])
  f(uj)3 : Subsystem  TreatAsAtomicUnit=on  mask{slope=sigslopef, offset=0.5}
      mask help: Created by Han, Cheol
      mask Display: plot([10 15 20 25 30 35 40 45 50], [0 0.01 0.1 0.2 0.5 0.8 0.9 0.99 1])
  f(uj)4 : Subsystem  TreatAsAtomicUnit=on  mask{slope=sigslopef, offset=0.5}
      mask help: Created by Han, Cheol
      mask Display: plot([10 15 20 25 30 35 40 45 50], [0 0.01 0.1 0.2 0.5 0.8 0.9 0.99 1])
  f(uj)5 : Subsystem  TreatAsAtomicUnit=on  mask{slope=sigslopef, offset=0.5}
      mask help: Created by Han, Cheol
      mask Display: plot([10 15 20 25 30 35 40 45 50], [0 0.01 0.1 0.2 0.5 0.8 0.9 0.99 1])
  p{1..20} (20 alike) : Product  RndMeth=Zero
  s{1..5} (5 alike) : Sum  Inputs=+++++
  Iu1,Iu2,Iu3,Iu4,Iu5 : Outport
  sij weights : Outport  Port=2
  sij weights1 : Outport  Port=3
  sij weights2 : Outport  Port=4
  wires:
  Demux/1 -> 15/1(ui), 45/1(ui), 35/1(ui), 25/1(ui), 5/1(ui)
  Demux/2 -> 4/1(ui), 44/1(ui), 34/1(ui), 24/1(ui), 14/1(ui)
  Demux/3 -> 43/1(ui), 33/1(ui), 23/1(ui), 13/1(ui), 3/1(ui)
  Demux/4 -> 42/1(ui), 32/1(ui), 22/1(ui), 12/1(ui), " 2"/1(ui)
  Demux/5 -> 41/1(ui), 31/1(ui), 21/1(ui), 11/1(ui), " "/1(ui)
  Demux1/1 -> " "/2(uj), " 2"/2(uj), 3/2(uj), 4/2(uj), 5/2(uj), f(uj)3/1(x)
  Demux1/2 -> 11/2(uj), 12/2(uj), 13/2(uj), 14/2(uj), 15/2(uj), f(uj)1/1(x)
  Demux1/3 -> 25/2(uj), 21/2(uj), 22/2(uj), 23/2(uj), 24/2(uj), f(uj)2/1(x)
  Demux1/4 -> 31/2(uj), 32/2(uj), 33/2(uj), 34/2(uj), 35/2(uj), f(uj)4/1(x)
  Demux1/5 -> 42/2(uj), 41/2(uj), f(uj)5/1(x), 43/2(uj), 44/2(uj), 45/2(uj)
  " "/1(Out1) -> Product/1, Mux1/5
  11/1(Out1) -> Product1/2, Mux1/4
  41/1(Out1) -> Product4/2, Mux1/1
  21/1(Out1) -> Product2/1, Mux1/3
  31/1(Out1) -> Product3/1, Mux1/2
  f(uj)3/1(y) -> Product/2, p5/2, p9/2, p15/1, p20/2
  f(uj)1/1(y) -> Product1/1, p4/2, p8/2, p14/1, p19/2  "uj2"
  f(uj)2/1(y) -> Product2/2, p3/2, p7/2, p13/1, p18/2  "uj3"
  f(uj)4/1(y) -> Product3/2, p2/2, p6/2, p17/2, p12/1
  " 2"/1(Out1) -> p5/1
  12/1(Out1) -> p4/1
  22/1(Out1) -> p3/1
  32/1(Out1) -> p2/1
  42/1(Out1) -> p1/2
  f(uj)5/1(y) -> Product4/1, p1/1, p10/2, p11/1, p16/2
  5/1(Out1) -> p9/1
  15/1(Out1) -> p8/1
  25/1(Out1) -> p7/1
  35/1(Out1) -> p6/1
  45/1(Out1) -> p10/1
  3/1(Out1) -> p15/2, Mux3/1
  13/1(Out1) -> p14/2, Mux3/2
  23/1(Out1) -> p13/2, Mux3/3
  33/1(Out1) -> p12/2, Mux3/4
  43/1(Out1) -> p11/2, Mux3/5
  p15/1 -> s4/5
  p11/1 -> s4/1
  p12/1 -> s4/2
  p13/1 -> s4/3
  p14/1 -> s4/4
  UI/1 -> Demux/1
  4/1(Out1) -> p20/1, Mux2/5
  SIJ/1 -> 41/3(Sij), 21/3(Sij), 11/3(Sij), " "/3(Sij), " 2"/3(Sij), 3/3(Sij), 4/3(Sij), 5/3(Sij), 13/3(Sij), 14/3(Sij), 15/3(Sij), 12/3(Sij), 22/3(Sij), 23/3(Sij), 24/3(Sij), 25/3(Sij), 31/3(Sij), 33/3(Sij), 34/3(Sij), 35/3(Sij), 32/3(Sij), 42/3(Sij), 43/3(Sij), 44/3(Sij), 45/3(Sij)
  14/1(Out1) -> p19/1, Mux2/4
  24/1(Out1) -> p18/1, Mux2/3
  UJ/1 -> Demux1/1
  34/1(Out1) -> p17/1, Mux2/2
  44/1(Out1) -> p16/1, Mux2/1
  Product/1 -> s1/5
  Product1/1 -> s1/4
  Product2/1 -> s1/3
  Product3/1 -> s1/2
  Product4/1 -> s1/1
  p1/1 -> s2/1
  p10/1 -> s3/1
  p2/1 -> s2/2
  p3/1 -> s2/3
  p4/1 -> s2/4
  p5/1 -> s2/5
  p6/1 -> s3/2
  p7/1 -> s3/3
  p8/1 -> s3/4
  p9/1 -> s3/5
  p16/1 -> s5/1
  p17/1 -> s5/2
  p18/1 -> s5/3
  p19/1 -> s5/4
  p20/1 -> s5/5
  s4/1 -> Mux/3
  s1/1 -> Mux/1
  s2/1 -> Mux/2
  s3/1 -> Mux/5
  s5/1 -> Mux/4
  Mux/1 -> Iu1,Iu2,Iu3,Iu4,Iu5/1
  Mux1/1 -> sij weights/1
  Mux2/1 -> sij weights1/1
  Mux3/1 -> sij weights2/1

== system neuronchainv6/Subsystem ==
  Product : Product  RndMeth=Zero
  Saturation : Saturate  UpperLimit=1  LowerLimit=0
  Signal Generator : SignalGenerator  WaveForm=square  Frequency=0.25
  Sum : Sum  Inputs=|+-
  motoract vis inputs : Subsystem
  Out1 : Outport
  Out2 : Outport  Port=2
  Out3 : Outport  Port=3
  Out4 : Outport  Port=4
  wires:
  motoract vis inputs/1(Out1) -> Out1/1
  motoract vis inputs/2(Out2) -> Product/1, Sum/1, Out2/1
  Signal Generator/1 -> Product/2
  Product/1 -> Sum/2, Saturation/1
  Sum/1 -> Out4/1
  Saturation/1 -> Out3/1

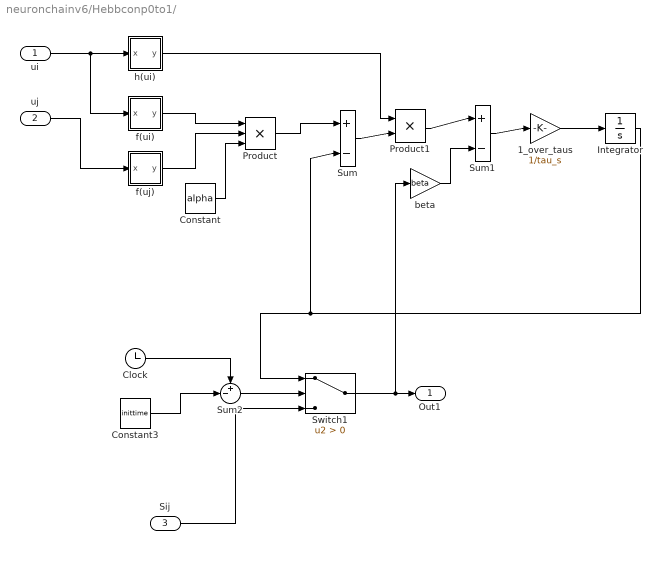
== system neuronchainv6/Hebbconp0to1/  ==
  ui : Inport
  uj : Inport  Port=2
  Sij : Inport  Port=3
  1_over_taus : Gain  Gain=1/tau_s
  Clock : Clock
      settings: Decimation=10
  Constant : Constant  Value=alpha
  Constant3 : Constant  Value=inittime
  Integrator : Integrator
  Product : Product  Inputs=3  RndMeth=Zero
  Product1 : Product  RndMeth=Zero
  Sum : Sum  Inputs=|+-
  Sum1 : Sum  Inputs=|+-
  Sum2 : Sum  Inputs=+-|
  Switch1 : Switch  Criteria=u2 > Threshold
  beta : Gain  Gain=beta
  f(ui) : Subsystem  TreatAsAtomicUnit=on  mask{slope=sigslopef, offset=0.5}
      mask help: Created by Han, Cheol
      mask Display: plot([10 15 20 25 30 35 40 45 50], [0 0.01 0.1 0.2 0.5 0.8 0.9 0.99 1])
  f(uj) : Subsystem  TreatAsAtomicUnit=on  mask{slope=sigslopef, offset=0.5}
      mask help: Created by Han, Cheol
      mask Display: plot([10 15 20 25 30 35 40 45 50], [0 0.01 0.1 0.2 0.5 0.8 0.9 0.99 1])
  h(ui) : Subsystem  TreatAsAtomicUnit=on  mask{slope=sigslopei, offset=0.5}
      mask help: Created by Han, Cheol
      mask Display: plot([10 15 20 25 30 35 40 45 50], [0 0.01 0.1 0.2 0.5 0.8 0.9 0.99 1])
  Out1 : Outport
  wires:
  ui/1 -> h(ui)/1(x), f(ui)/1(x)
  uj/1 -> f(uj)/1(x)
  f(ui)/1(y) -> Product/1
  f(uj)/1(y) -> Product/2
  Constant/1 -> Product/3
  Product/1 -> Sum/1
  Sum/1 -> Product1/2
  h(ui)/1(y) -> Product1/1
  Product1/1 -> Sum1/1
  beta/1 -> Sum1/2
  Sum1/1 -> 1_over_taus/1
  1_over_taus/1 -> Integrator/1
  Integrator/1 -> Switch1/1, Sum/2
  Sum2/1 -> Switch1/2
  Clock/1 -> Sum2/1
  Constant3/1 -> Sum2/2
  Switch1/1 -> beta/1, Out1/1
  Sij/1 -> Switch1/3

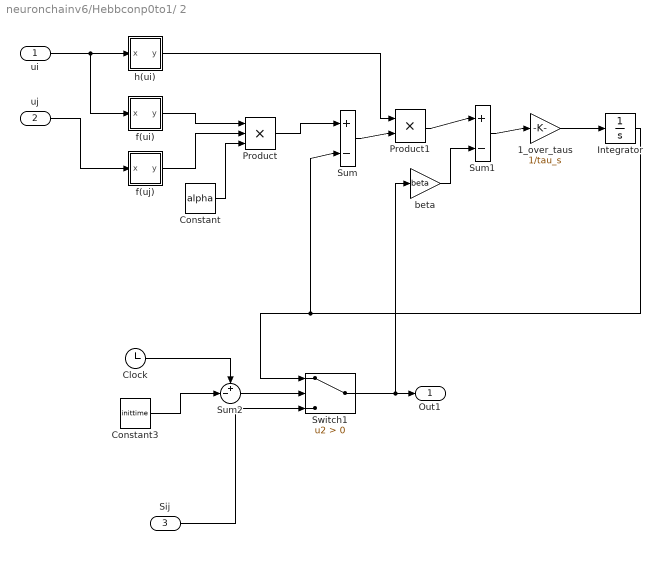
== system neuronchainv6/Hebbconp0to1/ 2 ==
  ui : Inport
  uj : Inport  Port=2
  Sij : Inport  Port=3
  1_over_taus : Gain  Gain=1/tau_s
  Clock : Clock
      settings: Decimation=10
  Constant : Constant  Value=alpha
  Constant3 : Constant  Value=inittime
  Integrator : Integrator
  Product : Product  Inputs=3  RndMeth=Zero
  Product1 : Product  RndMeth=Zero
  Sum : Sum  Inputs=|+-
  Sum1 : Sum  Inputs=|+-
  Sum2 : Sum  Inputs=+-|
  Switch1 : Switch  Criteria=u2 > Threshold
  beta : Gain  Gain=beta
  f(ui) : Subsystem  TreatAsAtomicUnit=on  mask{slope=sigslopef, offset=0.5}
      mask help: Created by Han, Cheol
      mask Display: plot([10 15 20 25 30 35 40 45 50], [0 0.01 0.1 0.2 0.5 0.8 0.9 0.99 1])
  f(uj) : Subsystem  TreatAsAtomicUnit=on  mask{slope=sigslopef, offset=0.5}
      mask help: Created by Han, Cheol
      mask Display: plot([10 15 20 25 30 35 40 45 50], [0 0.01 0.1 0.2 0.5 0.8 0.9 0.99 1])
  h(ui) : Subsystem  TreatAsAtomicUnit=on  mask{slope=sigslopei, offset=0.5}
      mask help: Created by Han, Cheol
      mask Display: plot([10 15 20 25 30 35 40 45 50], [0 0.01 0.1 0.2 0.5 0.8 0.9 0.99 1])
  Out1 : Outport
  wires:
  ui/1 -> h(ui)/1(x), f(ui)/1(x)
  uj/1 -> f(uj)/1(x)
  f(ui)/1(y) -> Product/1
  f(uj)/1(y) -> Product/2
  Constant/1 -> Product/3
  Product/1 -> Sum/1
  Sum/1 -> Product1/2
  h(ui)/1(y) -> Product1/1
  Product1/1 -> Sum1/1
  beta/1 -> Sum1/2
  Sum1/1 -> 1_over_taus/1
  1_over_taus/1 -> Integrator/1
  Integrator/1 -> Switch1/1, Sum/2
  Sum2/1 -> Switch1/2
  Clock/1 -> Sum2/1
  Constant3/1 -> Sum2/2
  Switch1/1 -> beta/1, Out1/1
  Sij/1 -> Switch1/3

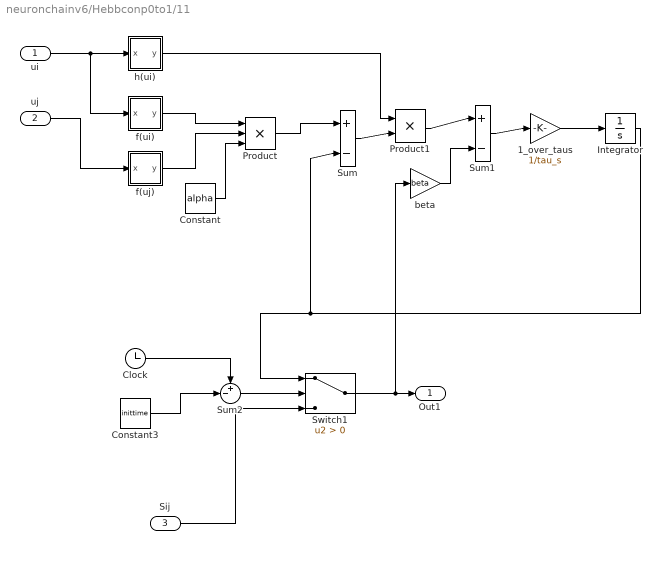
== system neuronchainv6/Hebbconp0to1/11 ==
  ui : Inport
  uj : Inport  Port=2
  Sij : Inport  Port=3
  1_over_taus : Gain  Gain=1/tau_s
  Clock : Clock
      settings: Decimation=10
  Constant : Constant  Value=alpha
  Constant3 : Constant  Value=inittime
  Integrator : Integrator
  Product : Product  Inputs=3  RndMeth=Zero
  Product1 : Product  RndMeth=Zero
  Sum : Sum  Inputs=|+-
  Sum1 : Sum  Inputs=|+-
  Sum2 : Sum  Inputs=+-|
  Switch1 : Switch  Criteria=u2 > Threshold
  beta : Gain  Gain=beta
  f(ui) : Subsystem  TreatAsAtomicUnit=on  mask{slope=sigslopef, offset=0.5}
      mask help: Created by Han, Cheol
      mask Display: plot([10 15 20 25 30 35 40 45 50], [0 0.01 0.1 0.2 0.5 0.8 0.9 0.99 1])
  f(uj) : Subsystem  TreatAsAtomicUnit=on  mask{slope=sigslopef, offset=0.5}
      mask help: Created by Han, Cheol
      mask Display: plot([10 15 20 25 30 35 40 45 50], [0 0.01 0.1 0.2 0.5 0.8 0.9 0.99 1])
  h(ui) : Subsystem  TreatAsAtomicUnit=on  mask{slope=sigslopei, offset=0.5}
      mask help: Created by Han, Cheol
      mask Display: plot([10 15 20 25 30 35 40 45 50], [0 0.01 0.1 0.2 0.5 0.8 0.9 0.99 1])
  Out1 : Outport
  wires:
  ui/1 -> h(ui)/1(x), f(ui)/1(x)
  uj/1 -> f(uj)/1(x)
  f(ui)/1(y) -> Product/1
  f(uj)/1(y) -> Product/2
  Constant/1 -> Product/3
  Product/1 -> Sum/1
  Sum/1 -> Product1/2
  h(ui)/1(y) -> Product1/1
  Product1/1 -> Sum1/1
  beta/1 -> Sum1/2
  Sum1/1 -> 1_over_taus/1
  1_over_taus/1 -> Integrator/1
  Integrator/1 -> Switch1/1, Sum/2
  Sum2/1 -> Switch1/2
  Clock/1 -> Sum2/1
  Constant3/1 -> Sum2/2
  Switch1/1 -> beta/1, Out1/1
  Sij/1 -> Switch1/3

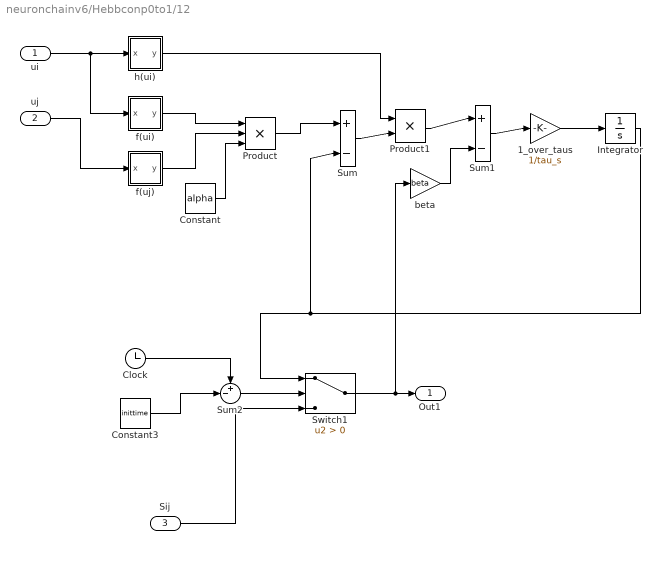
== system neuronchainv6/Hebbconp0to1/12 ==
  ui : Inport
  uj : Inport  Port=2
  Sij : Inport  Port=3
  1_over_taus : Gain  Gain=1/tau_s
  Clock : Clock
      settings: Decimation=10
  Constant : Constant  Value=alpha
  Constant3 : Constant  Value=inittime
  Integrator : Integrator
  Product : Product  Inputs=3  RndMeth=Zero
  Product1 : Product  RndMeth=Zero
  Sum : Sum  Inputs=|+-
  Sum1 : Sum  Inputs=|+-
  Sum2 : Sum  Inputs=+-|
  Switch1 : Switch  Criteria=u2 > Threshold
  beta : Gain  Gain=beta
  f(ui) : Subsystem  TreatAsAtomicUnit=on  mask{slope=sigslopef, offset=0.5}
      mask help: Created by Han, Cheol
      mask Display: plot([10 15 20 25 30 35 40 45 50], [0 0.01 0.1 0.2 0.5 0.8 0.9 0.99 1])
  f(uj) : Subsystem  TreatAsAtomicUnit=on  mask{slope=sigslopef, offset=0.5}
      mask help: Created by Han, Cheol
      mask Display: plot([10 15 20 25 30 35 40 45 50], [0 0.01 0.1 0.2 0.5 0.8 0.9 0.99 1])
  h(ui) : Subsystem  TreatAsAtomicUnit=on  mask{slope=sigslopei, offset=0.5}
      mask help: Created by Han, Cheol
      mask Display: plot([10 15 20 25 30 35 40 45 50], [0 0.01 0.1 0.2 0.5 0.8 0.9 0.99 1])
  Out1 : Outport
  wires:
  ui/1 -> h(ui)/1(x), f(ui)/1(x)
  uj/1 -> f(uj)/1(x)
  f(ui)/1(y) -> Product/1
  f(uj)/1(y) -> Product/2
  Constant/1 -> Product/3
  Product/1 -> Sum/1
  Sum/1 -> Product1/2
  h(ui)/1(y) -> Product1/1
  Product1/1 -> Sum1/1
  beta/1 -> Sum1/2
  Sum1/1 -> 1_over_taus/1
  1_over_taus/1 -> Integrator/1
  Integrator/1 -> Switch1/1, Sum/2
  Sum2/1 -> Switch1/2
  Clock/1 -> Sum2/1
  Constant3/1 -> Sum2/2
  Switch1/1 -> beta/1, Out1/1
  Sij/1 -> Switch1/3

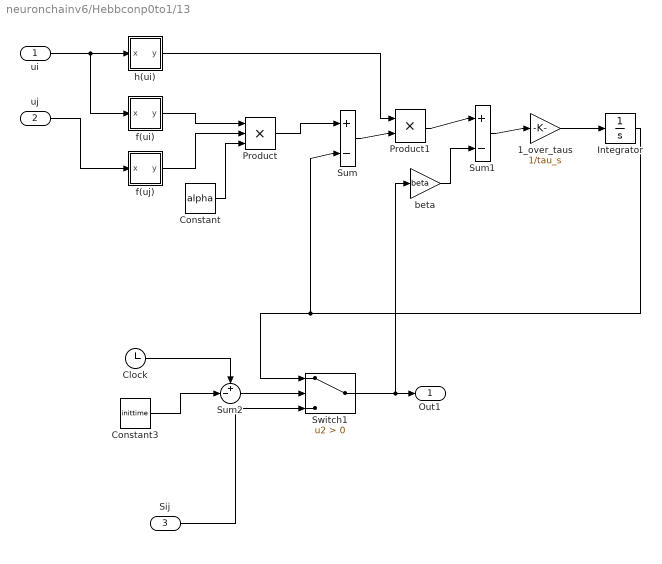
== system neuronchainv6/Hebbconp0to1/13 ==
  ui : Inport
  uj : Inport  Port=2
  Sij : Inport  Port=3
  1_over_taus : Gain  Gain=1/tau_s
  Clock : Clock
      settings: Decimation=10
  Constant : Constant  Value=alpha
  Constant3 : Constant  Value=inittime
  Integrator : Integrator
  Product : Product  Inputs=3  RndMeth=Zero
  Product1 : Product  RndMeth=Zero
  Sum : Sum  Inputs=|+-
  Sum1 : Sum  Inputs=|+-
  Sum2 : Sum  Inputs=+-|
  Switch1 : Switch  Criteria=u2 > Threshold
  beta : Gain  Gain=beta
  f(ui) : Subsystem  TreatAsAtomicUnit=on  mask{slope=sigslopef, offset=0.5}
      mask help: Created by Han, Cheol
      mask Display: plot([10 15 20 25 30 35 40 45 50], [0 0.01 0.1 0.2 0.5 0.8 0.9 0.99 1])
  f(uj) : Subsystem  TreatAsAtomicUnit=on  mask{slope=sigslopef, offset=0.5}
      mask help: Created by Han, Cheol
      mask Display: plot([10 15 20 25 30 35 40 45 50], [0 0.01 0.1 0.2 0.5 0.8 0.9 0.99 1])
  h(ui) : Subsystem  TreatAsAtomicUnit=on  mask{slope=sigslopei, offset=0.5}
      mask help: Created by Han, Cheol
      mask Display: plot([10 15 20 25 30 35 40 45 50], [0 0.01 0.1 0.2 0.5 0.8 0.9 0.99 1])
  Out1 : Outport
  wires:
  ui/1 -> h(ui)/1(x), f(ui)/1(x)
  uj/1 -> f(uj)/1(x)
  f(ui)/1(y) -> Product/1
  f(uj)/1(y) -> Product/2
  Constant/1 -> Product/3
  Product/1 -> Sum/1
  Sum/1 -> Product1/2
  h(ui)/1(y) -> Product1/1
  Product1/1 -> Sum1/1
  beta/1 -> Sum1/2
  Sum1/1 -> 1_over_taus/1
  1_over_taus/1 -> Integrator/1
  Integrator/1 -> Switch1/1, Sum/2
  Sum2/1 -> Switch1/2
  Clock/1 -> Sum2/1
  Constant3/1 -> Sum2/2
  Switch1/1 -> beta/1, Out1/1
  Sij/1 -> Switch1/3

== system neuronchainv6/Hebbconp0to1/14 ==
  ui : Inport
  uj : Inport  Port=2
  Sij : Inport  Port=3
  1_over_taus : Gain  Gain=1/tau_s
  Clock : Clock
      settings: Decimation=10
  Constant : Constant  Value=alpha
  Constant3 : Constant  Value=inittime
  Integrator : Integrator
  Product : Product  Inputs=3  RndMeth=Zero
  Product1 : Product  RndMeth=Zero
  Sum : Sum  Inputs=|+-
  Sum1 : Sum  Inputs=|+-
  Sum2 : Sum  Inputs=+-|
  Switch1 : Switch  Criteria=u2 > Threshold
  beta : Gain  Gain=beta
  f(ui) : Subsystem  TreatAsAtomicUnit=on  mask{slope=sigslopef, offset=0.5}
      mask help: Created by Han, Cheol
      mask Display: plot([10 15 20 25 30 35 40 45 50], [0 0.01 0.1 0.2 0.5 0.8 0.9 0.99 1])
  f(uj) : Subsystem  TreatAsAtomicUnit=on  mask{slope=sigslopef, offset=0.5}
      mask help: Created by Han, Cheol
      mask Display: plot([10 15 20 25 30 35 40 45 50], [0 0.01 0.1 0.2 0.5 0.8 0.9 0.99 1])
  h(ui) : Subsystem  TreatAsAtomicUnit=on  mask{slope=sigslopei, offset=0.5}
      mask help: Created by Han, Cheol
      mask Display: plot([10 15 20 25 30 35 40 45 50], [0 0.01 0.1 0.2 0.5 0.8 0.9 0.99 1])
  Out1 : Outport
  wires:
  ui/1 -> h(ui)/1(x), f(ui)/1(x)
  uj/1 -> f(uj)/1(x)
  f(ui)/1(y) -> Product/1
  f(uj)/1(y) -> Product/2
  Constant/1 -> Product/3
  Product/1 -> Sum/1
  Sum/1 -> Product1/2
  h(ui)/1(y) -> Product1/1
  Product1/1 -> Sum1/1
  beta/1 -> Sum1/2
  Sum1/1 -> 1_over_taus/1
  1_over_taus/1 -> Integrator/1
  Integrator/1 -> Switch1/1, Sum/2
  Sum2/1 -> Switch1/2
  Clock/1 -> Sum2/1
  Constant3/1 -> Sum2/2
  Switch1/1 -> beta/1, Out1/1
  Sij/1 -> Switch1/3

== system neuronchainv6/Hebbconp0to1/15 ==
  ui : Inport
  uj : Inport  Port=2
  Sij : Inport  Port=3
  1_over_taus : Gain  Gain=1/tau_s
  Clock : Clock
      settings: Decimation=10
  Constant : Constant  Value=alpha
  Constant3 : Constant  Value=inittime
  Integrator : Integrator
  Product : Product  Inputs=3  RndMeth=Zero
  Product1 : Product  RndMeth=Zero
  Sum : Sum  Inputs=|+-
  Sum1 : Sum  Inputs=|+-
  Sum2 : Sum  Inputs=+-|
  Switch1 : Switch  Criteria=u2 > Threshold
  beta : Gain  Gain=beta
  f(ui) : Subsystem  TreatAsAtomicUnit=on  mask{slope=sigslopef, offset=0.5}
      mask help: Created by Han, Cheol
      mask Display: plot([10 15 20 25 30 35 40 45 50], [0 0.01 0.1 0.2 0.5 0.8 0.9 0.99 1])
  f(uj) : Subsystem  TreatAsAtomicUnit=on  mask{slope=sigslopef, offset=0.5}
      mask help: Created by Han, Cheol
      mask Display: plot([10 15 20 25 30 35 40 45 50], [0 0.01 0.1 0.2 0.5 0.8 0.9 0.99 1])
  h(ui) : Subsystem  TreatAsAtomicUnit=on  mask{slope=sigslopei, offset=0.5}
      mask help: Created by Han, Cheol
      mask Display: plot([10 15 20 25 30 35 40 45 50], [0 0.01 0.1 0.2 0.5 0.8 0.9 0.99 1])
  Out1 : Outport
  wires:
  ui/1 -> h(ui)/1(x), f(ui)/1(x)
  uj/1 -> f(uj)/1(x)
  f(ui)/1(y) -> Product/1
  f(uj)/1(y) -> Product/2
  Constant/1 -> Product/3
  Product/1 -> Sum/1
  Sum/1 -> Product1/2
  h(ui)/1(y) -> Product1/1
  Product1/1 -> Sum1/1
  beta/1 -> Sum1/2
  Sum1/1 -> 1_over_taus/1
  1_over_taus/1 -> Integrator/1
  Integrator/1 -> Switch1/1, Sum/2
  Sum2/1 -> Switch1/2
  Clock/1 -> Sum2/1
  Constant3/1 -> Sum2/2
  Switch1/1 -> beta/1, Out1/1
  Sij/1 -> Switch1/3

== system neuronchainv6/Hebbconp0to1/21 ==
  ui : Inport
  uj : Inport  Port=2
  Sij : Inport  Port=3
  1_over_taus : Gain  Gain=1/tau_s
  Clock : Clock
      settings: Decimation=10
  Constant : Constant  Value=alpha
  Constant3 : Constant  Value=inittime
  Integrator : Integrator
  Product : Product  Inputs=3  RndMeth=Zero
  Product1 : Product  RndMeth=Zero
  Sum : Sum  Inputs=|+-
  Sum1 : Sum  Inputs=|+-
  Sum2 : Sum  Inputs=+-|
  Switch1 : Switch  Criteria=u2 > Threshold
  beta : Gain  Gain=beta
  f(ui) : Subsystem  TreatAsAtomicUnit=on  mask{slope=sigslopef, offset=0.5}
      mask help: Created by Han, Cheol
      mask Display: plot([10 15 20 25 30 35 40 45 50], [0 0.01 0.1 0.2 0.5 0.8 0.9 0.99 1])
  f(uj) : Subsystem  TreatAsAtomicUnit=on  mask{slope=sigslopef, offset=0.5}
      mask help: Created by Han, Cheol
      mask Display: plot([10 15 20 25 30 35 40 45 50], [0 0.01 0.1 0.2 0.5 0.8 0.9 0.99 1])
  h(ui) : Subsystem  TreatAsAtomicUnit=on  mask{slope=sigslopei, offset=0.5}
      mask help: Created by Han, Cheol
      mask Display: plot([10 15 20 25 30 35 40 45 50], [0 0.01 0.1 0.2 0.5 0.8 0.9 0.99 1])
  Out1 : Outport
  wires:
  ui/1 -> h(ui)/1(x), f(ui)/1(x)
  uj/1 -> f(uj)/1(x)
  f(ui)/1(y) -> Product/1
  f(uj)/1(y) -> Product/2
  Constant/1 -> Product/3
  Product/1 -> Sum/1
  Sum/1 -> Product1/2
  h(ui)/1(y) -> Product1/1
  Product1/1 -> Sum1/1
  beta/1 -> Sum1/2
  Sum1/1 -> 1_over_taus/1
  1_over_taus/1 -> Integrator/1
  Integrator/1 -> Switch1/1, Sum/2
  Sum2/1 -> Switch1/2
  Clock/1 -> Sum2/1
  Constant3/1 -> Sum2/2
  Switch1/1 -> beta/1, Out1/1
  Sij/1 -> Switch1/3

== system neuronchainv6/Hebbconp0to1/22 ==
  ui : Inport
  uj : Inport  Port=2
  Sij : Inport  Port=3
  1_over_taus : Gain  Gain=1/tau_s
  Clock : Clock
      settings: Decimation=10
  Constant : Constant  Value=alpha
  Constant3 : Constant  Value=inittime
  Integrator : Integrator
  Product : Product  Inputs=3  RndMeth=Zero
  Product1 : Product  RndMeth=Zero
  Sum : Sum  Inputs=|+-
  Sum1 : Sum  Inputs=|+-
  Sum2 : Sum  Inputs=+-|
  Switch1 : Switch  Criteria=u2 > Threshold
  beta : Gain  Gain=beta
  f(ui) : Subsystem  TreatAsAtomicUnit=on  mask{slope=sigslopef, offset=0.5}
      mask help: Created by Han, Cheol
      mask Display: plot([10 15 20 25 30 35 40 45 50], [0 0.01 0.1 0.2 0.5 0.8 0.9 0.99 1])
  f(uj) : Subsystem  TreatAsAtomicUnit=on  mask{slope=sigslopef, offset=0.5}
      mask help: Created by Han, Cheol
      mask Display: plot([10 15 20 25 30 35 40 45 50], [0 0.01 0.1 0.2 0.5 0.8 0.9 0.99 1])
  h(ui) : Subsystem  TreatAsAtomicUnit=on  mask{slope=sigslopei, offset=0.5}
      mask help: Created by Han, Cheol
      mask Display: plot([10 15 20 25 30 35 40 45 50], [0 0.01 0.1 0.2 0.5 0.8 0.9 0.99 1])
  Out1 : Outport
  wires:
  ui/1 -> h(ui)/1(x), f(ui)/1(x)
  uj/1 -> f(uj)/1(x)
  f(ui)/1(y) -> Product/1
  f(uj)/1(y) -> Product/2
  Constant/1 -> Product/3
  Product/1 -> Sum/1
  Sum/1 -> Product1/2
  h(ui)/1(y) -> Product1/1
  Product1/1 -> Sum1/1
  beta/1 -> Sum1/2
  Sum1/1 -> 1_over_taus/1
  1_over_taus/1 -> Integrator/1
  Integrator/1 -> Switch1/1, Sum/2
  Sum2/1 -> Switch1/2
  Clock/1 -> Sum2/1
  Constant3/1 -> Sum2/2
  Switch1/1 -> beta/1, Out1/1
  Sij/1 -> Switch1/3
